simulink model "FOC_EasyVersion"  (R2021a)
settings: Solver=VariableStepAuto  StartTime=0.0  StopTime=1.5  MaxStep=1e-5  RelTol=1e-3
model workspace (MAT data in the model file):
  ARR = 3000
  Flux_Linkage = 0.00185
  Inductor = 7e-05
  Pole_Pairs = 7
  Resistance = 0.05
  Tpwm = 5e-05
  UDC = 48
  deadtime = 0
libraries: pid_lib x3, spsDCVoltageSourceLib x1, spsPermanentMagnetSynchronousMachineLib x1, simulink x1, spsUniversalBridgeLib x1, spsabctodq0Lib x1, spspowerguiLib x1
settings Model: Creator=86139  LastModifiedBy=86139
settings SolverCC: ZeroCrossAlgorithm=Adaptive
settings DebuggingCC: IgnoredZcDiagnostic=none

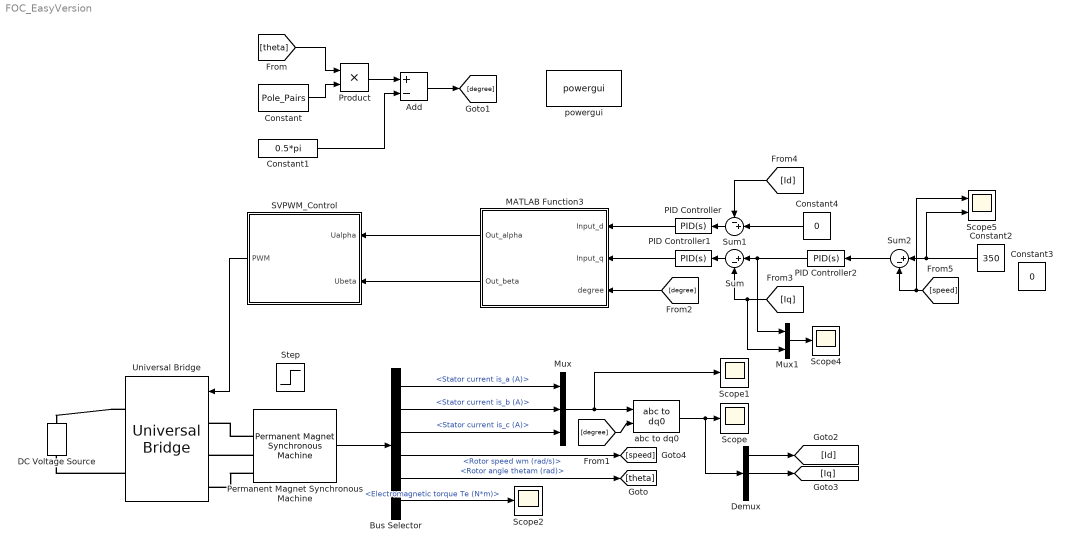
== system FOC_EasyVersion ==
  Add : Sum  Inputs=+-
  Bus Selector : BusSelector  OutputSignals=Stator current is_a (A),Stator current is_b (A),Stator current is_c (A),Rotor speed wm (rad/s),Rotor angle thetam (rad),Electromagnetic torque Te (N*m)
  Constant : Constant  Value=Pole_Pairs
  Constant1 : Constant  Value=0.5*pi
  Constant2 : Constant  Value=350
  Constant3 : Constant  Value=0
  Constant4 : Constant  Value=0
  DC Voltage Source : spsDCVoltageSourceLib/DC Voltage Source  Amplitude=UDC  Measurements=None
  Demux : Demux  Outputs=3
  MATLAB Function3 : MATLAB Function  TreatAsAtomicUnit=on
  Mux : Mux  Inputs=3
  Mux1 : Mux  Inputs=2
  PID Controller : pid_lib/PID Controller  Controller=PID  Form=Parallel  TimeDomain=Continuous-time  UseExternalTs=off  SampleTime=-1  IntegratorMethod=Forward Euler  FilterMethod=Forward Euler  ControllerParametersSource=internal  P=100  I=0  D=0  UseFilter=on  N=100  TunerSelectOption=Transfer Function Based (PID Tuner App)  InitialConditionSource=internal  InitialConditionForIntegrator=0  InitialConditionForFilter=0  DifferentiatorICPrevScaledInput=0  ExternalReset=none  TrackingMode=off  Kt=1  LimitOutput=off  SatLimitsSource=internal  UpperSaturationLimit=inf  LowerSaturationLimit=-inf  LinearizeAsGain=on  AntiWindupMode=none  Kb=1  POutMin=[]  POutMax=[]  IOutMin=[]  IOutMax=[]  DOutMin=[]  DOutMax=[]  NOutMin=[]  NOutMax=[]  SumOutMin=[]  SumOutMax=[]  SaturationOutMin=[]  SaturationOutMax=[]  PParamMin=[]  PParamMax=[]  IParamMin=[]  IParamMax=[]  DParamMin=[]  DParamMax=[]  NParamMin=[]  NParamMax=[]  KbParamMin=[]  KbParamMax=[]  KtParamMin=[]  KtParamMax=[]  KbOutMin=[]  KbOutMax=[]  KtOutMin=[]  KtOutMax=[]  IntegratorOutMin=[]  IntegratorOutMax=[]  FilterOutMin=[]  FilterOutMax=[]  SumI1OutMin=[]  SumI1OutMax=[]  SumI2OutMin=[]  SumI2OutMax=[]  SumI3OutMin=[]  SumI3OutMax=[]  SumI4OutMin=[]  SumI4OutMax=[]  SumDOutMin=[]  SumDOutMax=[]  DifferentiatorOutMin=[]  DifferentiatorOutMax=[]  FilterDiffOutCoefMin=[]  FilterDiffOutCoefMax=[]  ReciprocalOutMin=[]  ReciprocalOutMax=[]  SumDenOutMin=[]  SumDenOutMax=[]  SumNumOutMin=[]  SumNumOutMax=[]  DivideOutMin=[]  DivideOutMax=[]  UdiffTsProdOutMin=[]  UdiffTsProdOutMax=[]  NTsProdOutMin=[]  NTsProdOutMax=[]  UintegralTsProdOutMin=[]  UintegralTsProdOutMax=[]  UngainTsProdOutMin=[]  UngainTsProdOutMax=[]  IntegratorContinuousStateAttributes=''  IntegratorStateMustResolveToSignalObject=off  IntegratorRTWStateStorageClass=Auto  FilterContinuousStateAttributes=''  FilterStateMustResolveToSignalObject=off  FilterRTWStateStorageClass=Auto  ParallelPVariant=InternalParameters  IdealPVariant=Disabled  IVariant=InternalParameters  DVariant=InternalParameters  IntegratorVariant=Continuous  SatVariant=Disabled  AWVariant=Passthrough  PCopyVariant=Disabled  TRVariant=Disabled  FdbkBlocksVariant=Forward  IdealPFdbkVariant=Disabled  SatFdbkVariant=Disabled  DerivativeFilterVariant=ContFilter  NVariant=InternalParameters  NCopyVariant=Disabled  FilterICVariant=InternalICsFilter  IntegratorICVariant=InternalICs  ExternalResetVariant=Disabled  TRSumVariant=Passthrough  SumFdbkVariant=Disabled  SumVariant=Sum_PID  TsampFilterVariant=InternalTs  TsampNgainVariant=Passthrough  TsampIntegralVariant=Passthrough  ExternalSaturationOutDataTypeStr=Inherit: Same as second input
  PID Controller1 : pid_lib/PID Controller  Controller=PID  Form=Parallel  TimeDomain=Continuous-time  UseExternalTs=off  SampleTime=-1  IntegratorMethod=Forward Euler  FilterMethod=Forward Euler  ControllerParametersSource=internal  P=100  I=0  D=0  UseFilter=on  N=100  TunerSelectOption=Transfer Function Based (PID Tuner App)  InitialConditionSource=internal  InitialConditionForIntegrator=0  InitialConditionForFilter=0  DifferentiatorICPrevScaledInput=0  ExternalReset=none  TrackingMode=off  Kt=1  LimitOutput=off  SatLimitsSource=internal  UpperSaturationLimit=inf  LowerSaturationLimit=-inf  LinearizeAsGain=on  AntiWindupMode=none  Kb=1  POutMin=[]  POutMax=[]  IOutMin=[]  IOutMax=[]  DOutMin=[]  DOutMax=[]  NOutMin=[]  NOutMax=[]  SumOutMin=[]  SumOutMax=[]  SaturationOutMin=[]  SaturationOutMax=[]  PParamMin=[]  PParamMax=[]  IParamMin=[]  IParamMax=[]  DParamMin=[]  DParamMax=[]  NParamMin=[]  NParamMax=[]  KbParamMin=[]  KbParamMax=[]  KtParamMin=[]  KtParamMax=[]  KbOutMin=[]  KbOutMax=[]  KtOutMin=[]  KtOutMax=[]  IntegratorOutMin=[]  IntegratorOutMax=[]  FilterOutMin=[]  FilterOutMax=[]  SumI1OutMin=[]  SumI1OutMax=[]  SumI2OutMin=[]  SumI2OutMax=[]  SumI3OutMin=[]  SumI3OutMax=[]  SumI4OutMin=[]  SumI4OutMax=[]  SumDOutMin=[]  SumDOutMax=[]  DifferentiatorOutMin=[]  DifferentiatorOutMax=[]  FilterDiffOutCoefMin=[]  FilterDiffOutCoefMax=[]  ReciprocalOutMin=[]  ReciprocalOutMax=[]  SumDenOutMin=[]  SumDenOutMax=[]  SumNumOutMin=[]  SumNumOutMax=[]  DivideOutMin=[]  DivideOutMax=[]  UdiffTsProdOutMin=[]  UdiffTsProdOutMax=[]  NTsProdOutMin=[]  NTsProdOutMax=[]  UintegralTsProdOutMin=[]  UintegralTsProdOutMax=[]  UngainTsProdOutMin=[]  UngainTsProdOutMax=[]  IntegratorContinuousStateAttributes=''  IntegratorStateMustResolveToSignalObject=off  IntegratorRTWStateStorageClass=Auto  FilterContinuousStateAttributes=''  FilterStateMustResolveToSignalObject=off  FilterRTWStateStorageClass=Auto  ParallelPVariant=InternalParameters  IdealPVariant=Disabled  IVariant=InternalParameters  DVariant=InternalParameters  IntegratorVariant=Continuous  SatVariant=Disabled  AWVariant=Passthrough  PCopyVariant=Disabled  TRVariant=Disabled  FdbkBlocksVariant=Forward  IdealPFdbkVariant=Disabled  SatFdbkVariant=Disabled  DerivativeFilterVariant=ContFilter  NVariant=InternalParameters  NCopyVariant=Disabled  FilterICVariant=InternalICsFilter  IntegratorICVariant=InternalICs  ExternalResetVariant=Disabled  TRSumVariant=Passthrough  SumFdbkVariant=Disabled  SumVariant=Sum_PID  TsampFilterVariant=InternalTs  TsampNgainVariant=Passthrough  TsampIntegralVariant=Passthrough  ExternalSaturationOutDataTypeStr=Inherit: Same as second input
  PID Controller2 : pid_lib/PID Controller  Controller=PID  Form=Parallel  TimeDomain=Continuous-time  UseExternalTs=off  SampleTime=-1  IntegratorMethod=Forward Euler  FilterMethod=Forward Euler  ControllerParametersSource=internal  P=0.1  I=0  D=0  UseFilter=on  N=100  TunerSelectOption=Transfer Function Based (PID Tuner App)  InitialConditionSource=internal  InitialConditionForIntegrator=0  InitialConditionForFilter=0  DifferentiatorICPrevScaledInput=0  ExternalReset=none  TrackingMode=off  Kt=1  LimitOutput=on  SatLimitsSource=internal  UpperSaturationLimit=100  LowerSaturationLimit=-100  LinearizeAsGain=on  AntiWindupMode=none  Kb=1  POutMin=[]  POutMax=[]  IOutMin=[]  IOutMax=[]  DOutMin=[]  DOutMax=[]  NOutMin=[]  NOutMax=[]  SumOutMin=[]  SumOutMax=[]  SaturationOutMin=[]  SaturationOutMax=[]  PParamMin=[]  PParamMax=[]  IParamMin=[]  IParamMax=[]  DParamMin=[]  DParamMax=[]  NParamMin=[]  NParamMax=[]  KbParamMin=[]  KbParamMax=[]  KtParamMin=[]  KtParamMax=[]  KbOutMin=[]  KbOutMax=[]  KtOutMin=[]  KtOutMax=[]  IntegratorOutMin=[]  IntegratorOutMax=[]  FilterOutMin=[]  FilterOutMax=[]  SumI1OutMin=[]  SumI1OutMax=[]  SumI2OutMin=[]  SumI2OutMax=[]  SumI3OutMin=[]  SumI3OutMax=[]  SumI4OutMin=[]  SumI4OutMax=[]  SumDOutMin=[]  SumDOutMax=[]  DifferentiatorOutMin=[]  DifferentiatorOutMax=[]  FilterDiffOutCoefMin=[]  FilterDiffOutCoefMax=[]  ReciprocalOutMin=[]  ReciprocalOutMax=[]  SumDenOutMin=[]  SumDenOutMax=[]  SumNumOutMin=[]  SumNumOutMax=[]  DivideOutMin=[]  DivideOutMax=[]  UdiffTsProdOutMin=[]  UdiffTsProdOutMax=[]  NTsProdOutMin=[]  NTsProdOutMax=[]  UintegralTsProdOutMin=[]  UintegralTsProdOutMax=[]  UngainTsProdOutMin=[]  UngainTsProdOutMax=[]  IntegratorContinuousStateAttributes=''  IntegratorStateMustResolveToSignalObject=off  IntegratorRTWStateStorageClass=Auto  FilterContinuousStateAttributes=''  FilterStateMustResolveToSignalObject=off  FilterRTWStateStorageClass=Auto  ParallelPVariant=InternalParameters  IdealPVariant=Disabled  IVariant=InternalParameters  DVariant=InternalParameters  IntegratorVariant=Continuous  SatVariant=Enabled  AWVariant=Passthrough  PCopyVariant=Disabled  TRVariant=Disabled  FdbkBlocksVariant=Forward  IdealPFdbkVariant=Disabled  SatFdbkVariant=Disabled  DerivativeFilterVariant=ContFilter  NVariant=InternalParameters  NCopyVariant=Disabled  FilterICVariant=InternalICsFilter  IntegratorICVariant=InternalICs  ExternalResetVariant=Disabled  TRSumVariant=Passthrough  SumFdbkVariant=Disabled  SumVariant=Sum_PID  TsampFilterVariant=InternalTs  TsampNgainVariant=Passthrough  TsampIntegralVariant=Passthrough  ExternalSaturationOutDataTypeStr=Inherit: Same as second input
  Permanent Magnet Synchronous Machine : spsPermanentMagnetSynchronousMachineLib/Permanent Magnet Synchronous Machine  NbPhases=3  FluxDistribution=Sinusoidal  RotorType=Round  MechanicalLoad=Torque Tm  PresetModel=No  ShowDetailedParameters=on  MeasurementBus=off  Resistance=Resistance  Inductance=8.5e-3  dqInductances=[8.5e-3,8.5e-3]  La=Inductor  MachineConstant=Flux linkage established by magnets (V.s)  Flux=Flux_Linkage  VoltageCst=2.3489  TorqueCst=0.019425  Flat=120  Mechanical=[0.000127 0.0000004924 7 0]  PolePairs=4  InitialConditions=[0,0, 0,0]  InitialConditions5ph=[0 0 0 0 0 0]  RefAngle=90 degrees behind phase A axis (modified Park)  IterativeDiscreteModel=Trapezoidal non iterative  TsBlock=-1  TsPowergui=0
  Product : Product
  SVPWM_Control : Subsystem
  Scope{,1..2,4} (4 alike) : Scope
  Scope5 : Scope  NumInputPorts=2
  Step : Step  Time=0.1  SampleTime=0
  Sum : Sum  Inputs=|+-
  Sum1 : Sum  Inputs=-+|
  Sum2 : Sum  Inputs=|+-
  Universal Bridge : spsUniversalBridgeLib/Universal Bridge  Arms=3  SnubberResistance=1e5  SnubberCapacitance=inf  Device=MOSFET / Diodes  Ron=5e-4  Lon=0  ForwardVoltages="[  0  0  ]"  ForwardVoltage=0  GTOparameters=[ 10e-6 , 20e-6 ]  IGBTparameters=[ 1e-6 , 2e-6 ]  Measurements=None  Measurements_2=None  converterType=Rectifier
  abc to dq0 : spsabctodq0Lib/abc to dq0  Alignment=90 degrees behind phase A axis
  powergui : spspowerguiLib/powergui  Priority=1  SimulationMode=Continuous  SampleTime=50e-6  frequency=60  Iterations=50  frequencyindice=0  Pbase=100e6  ErrMax=1e-4  UnitsV=kV  UnitsW=MW  buscounter=0  FunctionMessages=off  echomessages=off  EnableUseOfTLC=off  CurrentSourceSwitches=off  DisableSnubberDevices=off  DisableRonSwitches=off  DisableVfSwitches=off  DisplayEquations=off  AutomaticDiscreteSolvers=off  SolverType=Tustin/Backward Euler (TBE)  Interpol=off  ExternalGateDelay=off  methode=off  Ts=100  x0status=blocks  SPID=on  SwTol=0  HookPort=off  NonlinearTolerance=1e-4  nMaxIteration=100  ContinueOnMaxIteration=off  RestoreLinks=warning  ResistiveCurrentMeasurement=off  Frange=[0:2:500]  Ylog=off  Xlog=on  ShowGrid=off  save=off  variable=ZData  structure=0  ZoomFFT=off  StartTime=0.0  cycles=1  DisplayStyle=1  fundamental=60  FreqAxis=off  MaxFrequency=1000  frequencyindicesteady=1  RmsSteady=1  display=off
  wires:
  Permanent Magnet Synchronous Machine/1 -> Bus Selector/1
  Bus Selector/1 -> Mux/1  "<Stator current is_a (A)>"
  Bus Selector/2 -> Mux/2  "<Stator current is_b (A)>"
  Bus Selector/3 -> Mux/3  "<Stator current is_c (A)>"
  Bus Selector/4 -> [speed]  "<Rotor speed wm (rad/s)>"
  Bus Selector/5 -> [theta]  "<Rotor angle thetam (rad)>"
  Bus Selector/6 -> Scope2/1  "<Electromagnetic torque Te (N*m)>"
  Mux/1 -> Scope1/1, abc to dq0/1
  [theta] -> Product/1
  Constant/1 -> Product/2
  Product/1 -> Add/1
  Constant1/1 -> Add/2
  Add/1 -> [degree]
  [degree] -> abc to dq0/2
  abc to dq0/1 -> Demux/1, Scope/1
  SVPWM_Control/1(PWM) -> Universal Bridge/1
  [degree] -> MATLAB Function3/3(degree)
  MATLAB Function3/1(Out_alpha) -> SVPWM_Control/1(Ualpha)
  MATLAB Function3/2(Out_beta) -> SVPWM_Control/2(Ubeta)
  Demux/2 -> [Iq]
  Sum1/1 -> PID Controller/1
  Sum/1 -> PID Controller1/1
  Constant4/1 -> Sum1/2
  PID Controller2/1 -> Mux1/1, Sum/1
  [speed] -> Scope5/1, Sum2/2
  Constant2/1 -> Scope5/2, Sum2/1
  Sum2/1 -> PID Controller2/1
  Demux/1 -> [Id]
  [Iq] -> Mux1/2, Sum/2
  [Id] -> Sum1/1
  PID Controller1/1 -> MATLAB Function3/2(Input_q)
  PID Controller/1 -> MATLAB Function3/1(Input_d)
  Mux1/1 -> Scope4/1
  connections:
  Permanent Magnet Synchronous Machine/LConn1 -- Universal Bridge/LConn1
  Permanent Magnet Synchronous Machine/LConn2 -- Universal Bridge/LConn2
  Permanent Magnet Synchronous Machine/LConn3 -- Universal Bridge/LConn3
  Universal Bridge/RConn1 -- DC Voltage Source/RConn1
  Universal Bridge/RConn2 -- DC Voltage Source/LConn1

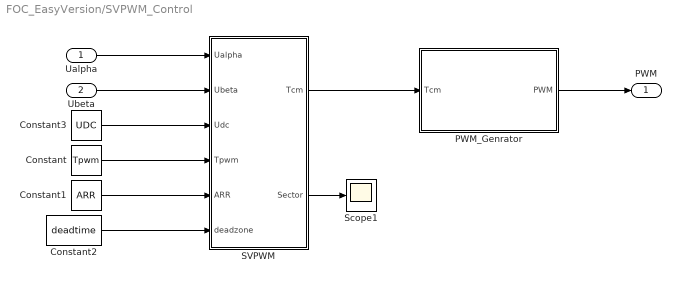
== system FOC_EasyVersion/SVPWM_Control ==
  Ualpha : Inport
  Ubeta : Inport  Port=2
  Constant : Constant  Value=Tpwm
  Constant1 : Constant  Value=ARR
  Constant2 : Constant  Value=deadtime
  Constant3 : Constant  Value=UDC
  PWM_Genrator : Subsystem
  SVPWM : Subsystem
  Scope1 : Scope
  PWM : Outport
  wires:
  Constant2/1 -> SVPWM/6(deadzone)
  Ualpha/1 -> SVPWM/1(Ualpha)
  Ubeta/1 -> SVPWM/2(Ubeta)
  Constant3/1 -> SVPWM/3(Udc)
  Constant/1 -> SVPWM/4(Tpwm)
  PWM_Genrator/1(PWM) -> PWM/1
  SVPWM/1(Tcm) -> PWM_Genrator/1(Tcm)
  Constant1/1 -> SVPWM/5(ARR)
  SVPWM/2(Sector) -> Scope1/1

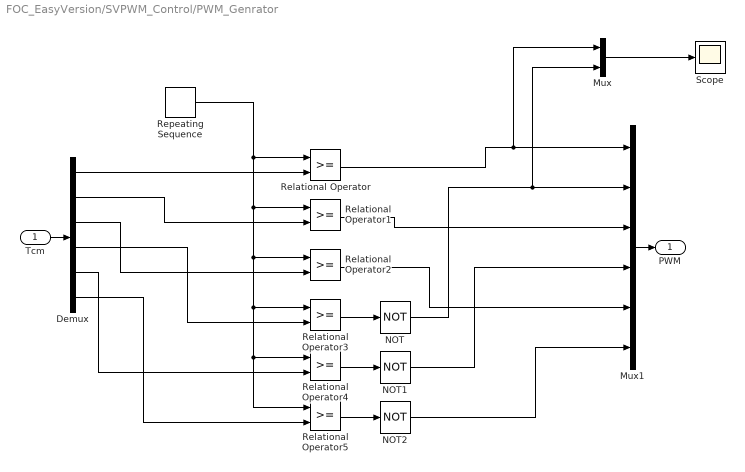
== system FOC_EasyVersion/SVPWM_Control/PWM_Genrator ==
  Tcm : Inport
  Demux : Demux  Outputs=6
  Mux : Mux  Inputs=2
  Mux1 : Mux  Inputs=6
  NOT : Logic  Operator=NOT  IconShape=distinctive  AllPortsSameDT=off  OutDataTypeStr=boolean
  NOT1 : Logic  Operator=NOT  IconShape=distinctive  AllPortsSameDT=off  OutDataTypeStr=boolean
  NOT2 : Logic  Operator=NOT  IconShape=distinctive  AllPortsSameDT=off  OutDataTypeStr=boolean
  Relational Operator{,1..5} (6 alike) : RelationalOperator  OutDataTypeStr=boolean  RndMeth=Simplest
  Repeating Sequence : simulink/Sources/Repeating Sequence  rep_seq_t=[0 0.5*Tpwm Tpwm]  rep_seq_y=[0 ARR 0]
  Scope : Scope
  PWM : Outport
  wires:
  Relational Operator4/1 -> NOT1/1
  Relational Operator5/1 -> NOT2/1
  Relational Operator/1 -> Mux/1, Mux1/1
  Demux/6 -> Relational Operator5/2
  Demux/4 -> Relational Operator3/2
  Repeating Sequence/1 -> Relational Operator5/1, Relational Operator4/1, Relational Operator3/1, Relational Operator2/1, Relational Operator1/1, Relational Operator/1
  Demux/2 -> Relational Operator1/2
  Demux/5 -> Relational Operator4/2
  Relational Operator3/1 -> NOT/1
  Mux1/1 -> PWM/1
  Demux/1 -> Relational Operator/2
  Demux/3 -> Relational Operator2/2
  Tcm/1 -> Demux/1
  NOT/1 -> Mux/2, Mux1/2
  Relational Operator1/1 -> Mux1/3
  Relational Operator2/1 -> Mux1/5
  NOT1/1 -> Mux1/4
  NOT2/1 -> Mux1/6
  Mux/1 -> Scope/1

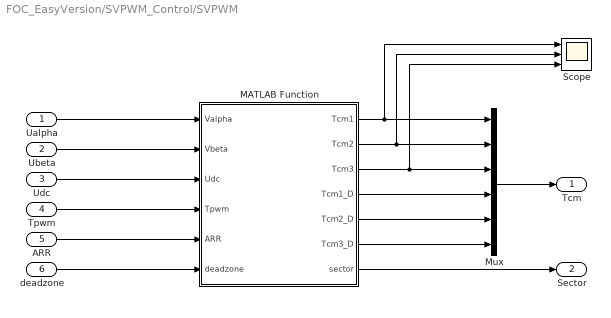
== system FOC_EasyVersion/SVPWM_Control/SVPWM ==
  Ualpha : Inport
  Ubeta : Inport  Port=2
  Udc : Inport  Port=3
  Tpwm : Inport  Port=4
  ARR : Inport  Port=5
  deadzone : Inport  Port=6
  MATLAB Function : MATLAB Function  TreatAsAtomicUnit=on
  Mux : Mux  Inputs=6
  Scope : Scope  NumInputPorts=3
  Tcm : Outport
  Sector : Outport  Port=2
  wires:
  Ualpha/1 -> MATLAB Function/1(Valpha)
  MATLAB Function/3(Tcm3) -> Scope/3, Mux/3
  Mux/1 -> Tcm/1
  MATLAB Function/2(Tcm2) -> Scope/2, Mux/2
  ARR/1 -> MATLAB Function/5(ARR)
  Tpwm/1 -> MATLAB Function/4(Tpwm)
  Udc/1 -> MATLAB Function/3(Udc)
  Ubeta/1 -> MATLAB Function/2(Vbeta)
  MATLAB Function/1(Tcm1) -> Scope/1, Mux/1
  MATLAB Function/7(sector) -> Sector/1
  deadzone/1 -> MATLAB Function/6(deadzone)
  MATLAB Function/4(Tcm1_D) -> Mux/4
  MATLAB Function/5(Tcm2_D) -> Mux/5
  MATLAB Function/6(Tcm3_D) -> Mux/6

== matlab function FOC_EasyVersion/SVPWM_Control/SVPWM/MATLAB Function ==
  data: Valpha input; Vbeta input; Tcm1 output; Tcm2 output; Tcm3 output; Tcm1_D output; Tcm2_D output; Tcm3_D output; sector output; Udc input; Tpwm input; ARR input; deadzone input
function [Tcm1,Tcm2,Tcm3,Tcm1_D,Tcm2_D,Tcm3_D,sector] = SVPWM(Valpha,Vbeta,Udc,Tpwm,ARR,deadzone)
%输出变量初始化
Tcm1 = 0;
Tcm2 = 0;
Tcm3 = 0;
sector = 0;


%扇区计算
%N与扇区对应的关系
%  3   1   5    4  6  2
%  I  II  III  IV  V  VI

Vref1 = Vbeta;
Vref2 = (sqrt(3)*Valpha-Vbeta)/2;
Vref3 = (-sqrt(3)*Valpha-Vbeta)/2;

if(Vref1>0)
    sector = 1;
end

if(Vref2>0)
    sector = sector+2;
end

if(Vref3>0)
    sector = sector+4;
end


%扇区内合成矢量作用时间计算
X = sqrt(3)*Vbeta*Tpwm/Udc;
Y = Tpwm/Udc*(3/2*Valpha+sqrt(3)/2*Vbeta);
Z = Tpwm/Udc*(-3/2*Valpha+sqrt(3)/2*Vbeta);

switch(sector)
    case 1
        T1 = Z;T2 = Y;
    case 2
        T1 = Y;T2 = -X;
    case 3
        T1 = -Z;T2 = X;
    case 4
        T1 = -X;T2 = Z;
    case 5
        T1 = X;T2 = -Y;
    otherwise
        T1 = -Y;T2 = -Z;
end

%过调制处理
if(T1+T2>Tpwm)
    T1 = Tpwm*T1/(T1+T2);
    T2 = Tpwm*T2/(T1+T2);
else
    T1 = T1;
    T2 = T2;
end


%扇区内合成矢量切换点时间计算
%此处为7段式，两个零矢量000 111 111插在中间，000均分插在两端
ta = (Tpwm-(T1+T2))/4;
tb = ta+T1/2;
tc = tb+T2/2;


%输出调制信号
switch(sector)
    case 1
        Tcm1 = tb;
        Tcm2 = ta;
        Tcm3 = tc;
    case 2
        Tcm1 = ta;
        Tcm2 = tc;
        Tcm3 = tb;
    case 3
        Tcm1 = ta;
        Tcm2 = tb;
        Tcm3 = tc;
    case 4
        Tcm1 = tc;
        Tcm2 = tb;
        Tcm3 = ta;
    case 5
        Tcm1 = tc;
        Tcm2 = ta;
        Tcm3 = tb;
    case 6
        Tcm1 = tb;
        Tcm2 = tc;
        Tcm3 = ta;
end


%调制信号处理，生成输入到MCU中的调制信号
Tcm1 = 2*Tcm1/Tpwm; 
Tcm2 = 2*Tcm2/Tpwm;
Tcm3 = 2*Tcm3/Tpwm;

Tcm1 = Tcm1*ARR; 
Tcm2 = Tcm2*ARR; 
Tcm3 = Tcm3*ARR;

Tcm1_D = Tcm1-deadzone;
Tcm2_D = Tcm2-deadzone;
Tcm3_D = Tcm3-deadzone;
%防止溢出
if(Tcm1_D<0)
    Tcm1_D=0;
end

if(Tcm2_D<0)
    Tcm2_D=0;
end

if(Tcm3_D<0)
    Tcm3_D=0;
end

end

== matlab function FOC_EasyVersion/MATLAB Function3 ==
  data: Input_d input; Out_alpha output; Input_q input; degree input; Out_beta output
function [Out_alpha,Out_beta]= Inverse_Park_transform(Input_d,Input_q,degree)
%反Park变换

Out_alpha=cos(degree)*Input_d-sin(degree)*Input_q;
Out_beta=sin(degree)*Input_d+cos(degree)*Input_q;

end
